simulink model "BLDC"  (R2024a)
settings: Solver=VariableStepAuto  StartTime=0.0  StopTime=10.0  RelTol=1e-3
libraries: c2838x_M4_lib x1
settings Model: Creator=d  LastModifiedBy=d

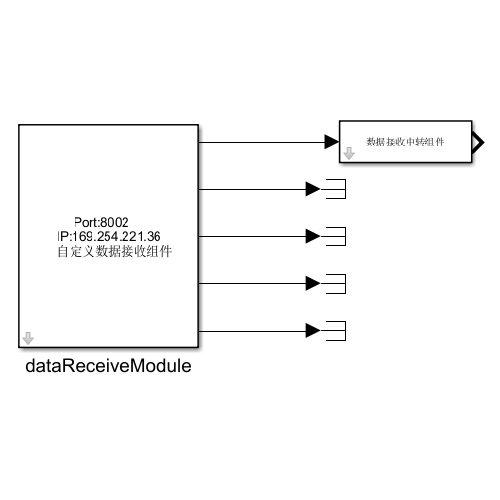
[thumbnail: Simulink's stored preview of the top-level diagram]
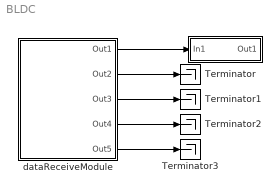
== system BLDC ==
  " " : Subsystem
      mask DialogControl ParameterGroupVar Prompt: 参数
  Terminator{,1..3} (4 alike) : Terminator
  dataReceiveModule : Subsystem
      mask DialogControl ParameterGroupVar Prompt: 参数
  wires:
  dataReceiveModule/2(Out2) -> Terminator/1
  dataReceiveModule/4(Out4) -> Terminator2/1
  dataReceiveModule/3(Out3) -> Terminator1/1
  dataReceiveModule/5(Out5) -> Terminator3/1
  dataReceiveModule/1(Out1) -> " "/1(In1)

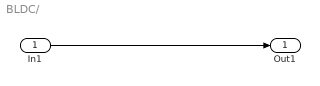
== system BLDC/  ==
  In1 : Inport
  Out1 : Outport
  wires:
  In1/1 -> Out1/1

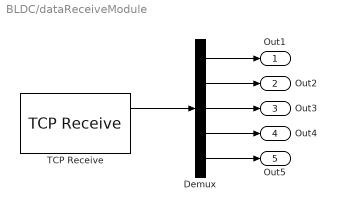
== system BLDC/dataReceiveModule ==
  Demux : Demux  Outputs=5
  TCP Receive : c2838x_M4_lib/TCP Receive  ConnectionMode=Server  RemoteIPAddress_=192.168.1.10  ServerIPPort_=25002  LocalIPPort_=25000  DataType=uint8  DataLength=1  BlockingMode=on  SampleTime=0.1
  Out1 : Outport
  Out2 : Outport  Port=2
  Out3 : Outport  Port=3
  Out4 : Outport  Port=4
  Out5 : Outport  Port=5
  wires:
  TCP Receive/1 -> Demux/1
  Demux/1 -> Out1/1
  Demux/2 -> Out2/1
  Demux/3 -> Out3/1
  Demux/4 -> Out4/1
  Demux/5 -> Out5/1
